simulink model "closed_loop_system_monitoring"  (R2025b)
settings: Solver=FixedStepAuto  StartTime=0.0  StopTime=2  RelTol=1e-3
values from neighbouring files (symbols this model uses):
  A = [Ac 0*Ac ... (first row only)    [closed_loop_system.m]
  B = [Bc ... (first row only)    [closed_loop_system.m]
  C = [0 0 Cp]    [closed_loop_system.m]
  Ts = 1/100    (= 0.01)    [closed_loop_system.m]
(part 2 of 2)

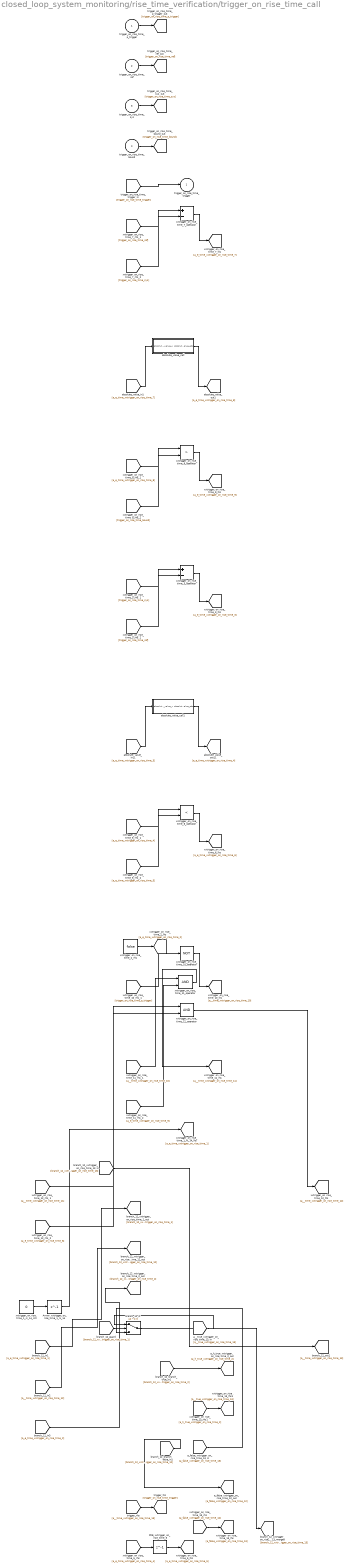
== system closed_loop_system_monitoring/rise_time_verification/trigger_on_rise_time_call ==
  trigger_on_rise_time_p_trigger : Inport  OutDataTypeStr=boolean
  trigger_on_rise_time_ref : Inport  Port=2  OutDataTypeStr=double
  trigger_on_rise_time_sys : Inport  Port=3  OutDataTypeStr=double
  trigger_on_rise_time_bound : Inport  Port=4  OutDataTypeStr=double
  Arrow_xxtrigger_on_rise_time_1_ni_14 : Delay  DelayLength=1  InitialCondition=1
  PRE_xxtrigger_on_rise_time_5 : Delay  DelayLength=1  InitialCondition=0
  absolute_value_call : Subsystem
  absolute_value_call1 : Subsystem
  branch_12_IF : Switch  Criteria=u2 ~= 0  SaturateOnIntegerOverflow=off  InputSameDT=off
  xxtrigger_on_rise_time_10_operator : Logic  Operator=NOT  AllPortsSameDT=off  OutDataTypeStr=boolean
  xxtrigger_on_rise_time_11_operator : Logic  AllPortsSameDT=off  OutDataTypeStr=boolean
  xxtrigger_on_rise_time_12_operator : Logic  AllPortsSameDT=off  OutDataTypeStr=boolean
  xxtrigger_on_rise_time_1_ni_14_init : Constant  Value=0  OutDataTypeStr=boolean
  xxtrigger_on_rise_time_2_rhs : Constant  Value=false  OutDataTypeStr=boolean
  xxtrigger_on_rise_time_3_operator : Sum  Inputs=+-  OutDataTypeStr=double
  xxtrigger_on_rise_time_6_operator : RelationalOperator  Operator=<  OutDataTypeStr=boolean  RndMeth=Simplest  InputSameDT=off
  xxtrigger_on_rise_time_7_operator : Sum  Inputs=+-  OutDataTypeStr=double
  xxtrigger_on_rise_time_9_operator : RelationalOperator  Operator=>  OutDataTypeStr=boolean  RndMeth=Simplest  InputSameDT=off
  trigger_on_rise_time_trigger : Outport
  wires:
  PRE_xxtrigger_on_rise_time_5/1 -> [a_e_time_xxtrigger_on_rise_time_5]
  [a_e_time_xxtrigger_on_rise_time_4] -> PRE_xxtrigger_on_rise_time_5/1
  [a__time_xxtrigger_on_rise_time_13] -> [trigger_on_rise_time_trigger]
  [branch_12_xxtrigger_on_rise_time_2] -> [a_h_true_xxtrigger_on_rise_time_2]
  [a_h_true_xxtrigger_on_rise_time_2] -> [a__true_xxtrigger_on_rise_time_13]
  [branch_12_xxtrigger_on_rise_time_12] -> [a_false_xxtrigger_on_rise_time_12]
  [a_false_xxtrigger_on_rise_time_12] -> [a_false_xxtrigger_on_rise_time_13]
  [a_e_time_xxtrigger_on_rise_time_1] -> [branch_12_xxtrigger_on_rise_time_1]
  [a__time_xxtrigger_on_rise_time_12] -> [branch_12_xxtrigger_on_rise_time_12]
  [a_e_time_xxtrigger_on_rise_time_2] -> [branch_12_xxtrigger_on_rise_time_2]
  [branch_12_xxtrigger_on_rise_time_1] -> branch_12_IF/2
  [a__true_xxtrigger_on_rise_time_13] -> branch_12_IF/1
  [a_false_xxtrigger_on_rise_time_13] -> branch_12_IF/3
  branch_12_IF/1 -> [branch_12_xxtrigger_on_rise_time_13]
  [branch_12_xxtrigger_on_rise_time_13] -> [a__time_xxtrigger_on_rise_time_13]
  Arrow_xxtrigger_on_rise_time_1_ni_14/1 -> [a_e_time_xxtrigger_on_rise_time_1]
  xxtrigger_on_rise_time_1_ni_14_init/1 -> Arrow_xxtrigger_on_rise_time_1_ni_14/1
  [a_e_time_xxtrigger_on_rise_time_6] -> xxtrigger_on_rise_time_12_operator/2
  [a__time_xxtrigger_on_rise_time_11] -> xxtrigger_on_rise_time_12_operator/1
  xxtrigger_on_rise_time_12_operator/1 -> [a__time_xxtrigger_on_rise_time_12]
  [a_e_time_xxtrigger_on_rise_time_9] -> xxtrigger_on_rise_time_11_operator/2
  [a__time_xxtrigger_on_rise_time_10] -> xxtrigger_on_rise_time_11_operator/1
  xxtrigger_on_rise_time_11_operator/1 -> [a__time_xxtrigger_on_rise_time_11]
  [trigger_on_rise_time_p_trigger] -> xxtrigger_on_rise_time_10_operator/1
  xxtrigger_on_rise_time_10_operator/1 -> [a__time_xxtrigger_on_rise_time_10]
  xxtrigger_on_rise_time_2_rhs/1 -> [a_e_time_xxtrigger_on_rise_time_2]
  [a_e_time_xxtrigger_on_rise_time_5] -> xxtrigger_on_rise_time_6_operator/2
  [a_e_time_xxtrigger_on_rise_time_4] -> xxtrigger_on_rise_time_6_operator/1
  xxtrigger_on_rise_time_6_operator/1 -> [a_e_time_xxtrigger_on_rise_time_6]
  [a_e_time_xxtrigger_on_rise_time_3] -> absolute_value_call1/1(absolute_value_x)
  absolute_value_call1/1(absolute_value_abs) -> [a_e_time_xxtrigger_on_rise_time_4]
  [trigger_on_rise_time_ref] -> xxtrigger_on_rise_time_3_operator/2
  [trigger_on_rise_time_sys] -> xxtrigger_on_rise_time_3_operator/1
  xxtrigger_on_rise_time_3_operator/1 -> [a_e_time_xxtrigger_on_rise_time_3]
  [trigger_on_rise_time_bound] -> xxtrigger_on_rise_time_9_operator/2
  [a_e_time_xxtrigger_on_rise_time_8] -> xxtrigger_on_rise_time_9_operator/1
  xxtrigger_on_rise_time_9_operator/1 -> [a_e_time_xxtrigger_on_rise_time_9]
  [a_e_time_xxtrigger_on_rise_time_7] -> absolute_value_call/1(absolute_value_x)
  absolute_value_call/1(absolute_value_abs) -> [a_e_time_xxtrigger_on_rise_time_8]
  [trigger_on_rise_time_sys] -> xxtrigger_on_rise_time_7_operator/2
  [trigger_on_rise_time_ref] -> xxtrigger_on_rise_time_7_operator/1
  xxtrigger_on_rise_time_7_operator/1 -> [a_e_time_xxtrigger_on_rise_time_7]
  [trigger_on_rise_time_trigger] -> trigger_on_rise_time_trigger/1
  trigger_on_rise_time_bound/1 -> [trigger_on_rise_time_bound]
  trigger_on_rise_time_sys/1 -> [trigger_on_rise_time_sys]
  trigger_on_rise_time_ref/1 -> [trigger_on_rise_time_ref]
  trigger_on_rise_time_p_trigger/1 -> [trigger_on_rise_time_p_trigger]

== system closed_loop_system_monitoring/rise_time_verification/eventually_false_var_call/forall_a_var_call ==
  forall_a_var_inside_time_interval : Inport  OutDataTypeStr=boolean
  forall_a_var_prop : Inport  Port=2  OutDataTypeStr=boolean
  exist_var_call : Subsystem
  output_operator : Logic  Operator=NOT  AllPortsSameDT=off  OutDataTypeStr=boolean
  xxforall_a_var_1_operator : Logic  Operator=NOT  AllPortsSameDT=off  OutDataTypeStr=boolean
  forall_a_var_output : Outport
  wires:
  forall_a_var_inside_time_interval/1 -> [forall_a_var_inside_time_interval]
  forall_a_var_prop/1 -> [forall_a_var_prop]
  [forall_a_var_output] -> forall_a_var_output/1
  xxforall_a_var_1_operator/1 -> [forall_a_var_xxforall_a_var_1]
  [forall_a_var_prop] -> xxforall_a_var_1_operator/1
  exist_var_call/1(exist_var_output) -> [forall_a_var_xxforall_a_var_2]
  [forall_a_var_inside_time_interval] -> exist_var_call/1(exist_var_inside_time_interval)
  [forall_a_var_xxforall_a_var_1] -> exist_var_call/2(exist_var_prop)
  output_operator/1 -> [forall_a_var_output]
  [forall_a_var_xxforall_a_var_2] -> output_operator/1

== system closed_loop_system_monitoring/rise_time_verification/eventually_false_var_call/min_call ==
  min_a : Inport
  min_b : Inport  Port=2
  branch_1_IF : Switch  Criteria=u2 ~= 0  SaturateOnIntegerOverflow=off  InputSameDT=off
  xxmin_1_operator : RelationalOperator  Operator=<=  OutDataTypeStr=boolean  RndMeth=Simplest  InputSameDT=off
  min_valeur_min : Outport
  wires:
  min_a/1 -> [min_a]
  min_b/1 -> [min_b]
  [min_valeur_min] -> min_valeur_min/1
  xxmin_1_operator/1 -> [min_xxmin_1]
  [min_a] -> xxmin_1_operator/1
  [min_b] -> xxmin_1_operator/2
  [branch_1_valeur_min] -> [min_valeur_min]
  branch_1_IF/1 -> [branch_1_valeur_min]
  [branch_1_branch_false_valeur_min] -> branch_1_IF/3
  [branch_1_branch_true_valeur_min] -> branch_1_IF/1
  [branch_1_xxmin_1] -> branch_1_IF/2
  [min_b] -> [branch_1_b]
  [min_a] -> [branch_1_a]
  [min_xxmin_1] -> [branch_1_xxmin_1]
  [branch_1_branch_false_b] -> [branch_1_branch_false_valeur_min]
  [branch_1_b] -> [branch_1_branch_false_b]
  [branch_1_branch_true_a] -> [branch_1_branch_true_valeur_min]
  [branch_1_a] -> [branch_1_branch_true_a]

== system closed_loop_system_monitoring/rise_time_verification/eventually_false_var_call/timeab_var_call ==
  timeab_var_a : Inport
  timeab_var_b : Inport  Port=2
  timeab_tmp_var_call : Subsystem
  timeab_var_inside_time_interval : Outport
  wires:
  timeab_var_a/1 -> [timeab_var_a]
  timeab_var_b/1 -> [timeab_var_b]
  [timeab_var_inside_time_interval] -> timeab_var_inside_time_interval/1
  timeab_tmp_var_call/1(timeab_tmp_var_internal_clk) -> [timeab_var_iclk]
  timeab_tmp_var_call/2(timeab_tmp_var_inside_time_interval) -> [timeab_var_inside_time_interval]
  [timeab_var_a] -> timeab_tmp_var_call/1(timeab_tmp_var_a)
  [timeab_var_b] -> timeab_tmp_var_call/2(timeab_tmp_var_b)

== system closed_loop_system_monitoring/rise_time_verification/eventually_true_var_call/exist_var_call ==
  exist_var_inside_time_interval : Inport  OutDataTypeStr=boolean
  exist_var_prop : Inport  Port=2  OutDataTypeStr=boolean
  output_operator : Logic  AllPortsSameDT=off  OutDataTypeStr=boolean
  exist_var_output : Outport
  wires:
  exist_var_inside_time_interval/1 -> [exist_var_inside_time_interval]
  exist_var_prop/1 -> [exist_var_prop]
  [exist_var_output] -> exist_var_output/1
  output_operator/1 -> [exist_var_output]
  [exist_var_inside_time_interval] -> output_operator/1
  [exist_var_prop] -> output_operator/2

== system closed_loop_system_monitoring/rise_time_verification/eventually_true_var_call/timeab_var_call ==
  timeab_var_a : Inport
  timeab_var_b : Inport  Port=2
  Scope : Scope  NumInputPorts=4
      settings: ActiveDisplayYMinimum=-0.12499999999999997  ActiveDisplayYMaximum=1.125  DataLoggingVariableName=ScopeData12
  timeab_tmp_var_call : Subsystem
  timeab_var_inside_time_interval : Outport
  wires:
  timeab_var_a/1 -> [timeab_var_a]
  timeab_var_b/1 -> [timeab_var_b]
  [timeab_var_inside_time_interval] -> timeab_var_inside_time_interval/1
  timeab_tmp_var_call/1(timeab_tmp_var_internal_clk) -> Scope/2, [timeab_var_iclk]
  timeab_tmp_var_call/2(timeab_tmp_var_inside_time_interval) -> Scope/1, [timeab_var_inside_time_interval]
  [timeab_var_a] -> Scope/3, timeab_tmp_var_call/1(timeab_tmp_var_a)
  [timeab_var_b] -> timeab_tmp_var_call/2(timeab_tmp_var_b), Scope/4

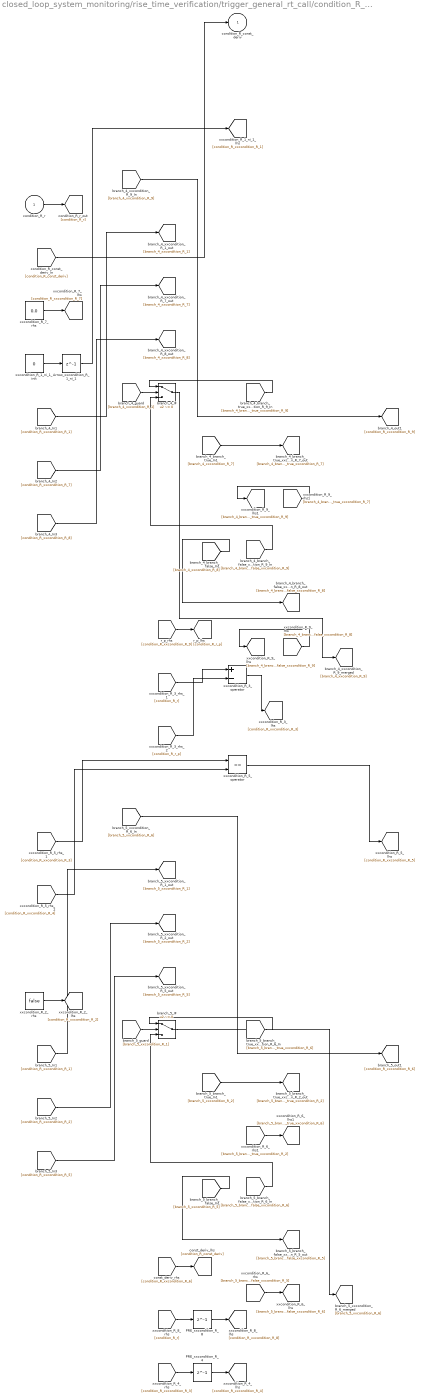
== system closed_loop_system_monitoring/rise_time_verification/trigger_general_rt_call/condition_R_call ==
  condition_R_r : Inport  OutDataTypeStr=double
  Arrow_xxcondition_R_1_ni_1 : Delay  DelayLength=1  InitialCondition=1
  PRE_xxcondition_R_4 : Delay  DelayLength=1  InitialCondition=0
  PRE_xxcondition_R_8 : Delay  DelayLength=1  InitialCondition=0
  branch_4_IF : Switch  Criteria=u2 ~= 0  SaturateOnIntegerOverflow=off  InputSameDT=off
  branch_5_IF : Switch  Criteria=u2 ~= 0  SaturateOnIntegerOverflow=off  InputSameDT=off
  xxcondition_R_1_ni_1_init : Constant  Value=0  OutDataTypeStr=boolean
  xxcondition_R_2_rhs : Constant  Value=false  OutDataTypeStr=boolean
  xxcondition_R_3_operator : Sum  Inputs=+-  OutDataTypeStr=double
  xxcondition_R_5_operator : RelationalOperator  Operator===  OutDataTypeStr=boolean  RndMeth=Simplest  InputSameDT=off
  xxcondition_R_7_rhs : Constant  Value=0.0  OutDataTypeStr=double
  condition_R_const_deriv : Outport
  wires:
  condition_R_r/1 -> [condition_R_r]
  [condition_R_const_deriv] -> condition_R_const_deriv/1
  xxcondition_R_7_rhs/1 -> [condition_R_xxcondition_R_7]
  xxcondition_R_1_ni_1_init/1 -> Arrow_xxcondition_R_1_ni_1/1
  Arrow_xxcondition_R_1_ni_1/1 -> [condition_R_xxcondition_R_1]
  [branch_4_xxcondition_R_9] -> [condition_R_xxcondition_R_9]
  branch_4_IF/1 -> [branch_4_xxcondition_R_9]
  [branch_4_branch_false_xxcondition_R_9] -> branch_4_IF/3
  [branch_4_branch_true_xxcondition_R_9] -> branch_4_IF/1
  [branch_4_xxcondition_R_1] -> branch_4_IF/2
  [condition_R_xxcondition_R_8] -> [branch_4_xxcondition_R_8]
  [condition_R_xxcondition_R_7] -> [branch_4_xxcondition_R_7]
  [condition_R_xxcondition_R_1] -> [branch_4_xxcondition_R_1]
  [branch_4_branch_false_xxcondition_R_8] -> [branch_4_branch_false_xxcondition_R_9]
  [branch_4_xxcondition_R_8] -> [branch_4_branch_false_xxcondition_R_8]
  [branch_4_branch_true_xxcondition_R_7] -> [branch_4_branch_true_xxcondition_R_9]
  [branch_4_xxcondition_R_7] -> [branch_4_branch_true_xxcondition_R_7]
  [condition_R_xxcondition_R_9] -> [condition_R_r_p]
  xxcondition_R_3_operator/1 -> [condition_R_xxcondition_R_3]
  [condition_R_r] -> xxcondition_R_3_operator/1
  [condition_R_r_p] -> xxcondition_R_3_operator/2
  xxcondition_R_5_operator/1 -> [condition_R_xxcondition_R_5]
  [condition_R_xxcondition_R_3] -> xxcondition_R_5_operator/1
  [condition_R_xxcondition_R_4] -> xxcondition_R_5_operator/2
  xxcondition_R_2_rhs/1 -> [condition_R_xxcondition_R_2]
  [branch_5_xxcondition_R_6] -> [condition_R_xxcondition_R_6]
  branch_5_IF/1 -> [branch_5_xxcondition_R_6]
  [branch_5_branch_false_xxcondition_R_6] -> branch_5_IF/3
  [branch_5_branch_true_xxcondition_R_6] -> branch_5_IF/1
  [branch_5_xxcondition_R_1] -> branch_5_IF/2
  [condition_R_xxcondition_R_5] -> [branch_5_xxcondition_R_5]
  [condition_R_xxcondition_R_2] -> [branch_5_xxcondition_R_2]
  [condition_R_xxcondition_R_1] -> [branch_5_xxcondition_R_1]
  [branch_5_branch_false_xxcondition_R_5] -> [branch_5_branch_false_xxcondition_R_6]
  [branch_5_xxcondition_R_5] -> [branch_5_branch_false_xxcondition_R_5]
  [branch_5_branch_true_xxcondition_R_2] -> [branch_5_branch_true_xxcondition_R_6]
  [branch_5_xxcondition_R_2] -> [branch_5_branch_true_xxcondition_R_2]
  [condition_R_xxcondition_R_6] -> [condition_R_const_deriv]
  [condition_R_r] -> PRE_xxcondition_R_8/1
  PRE_xxcondition_R_8/1 -> [condition_R_xxcondition_R_8]
  [condition_R_xxcondition_R_3] -> PRE_xxcondition_R_4/1
  PRE_xxcondition_R_4/1 -> [condition_R_xxcondition_R_4]

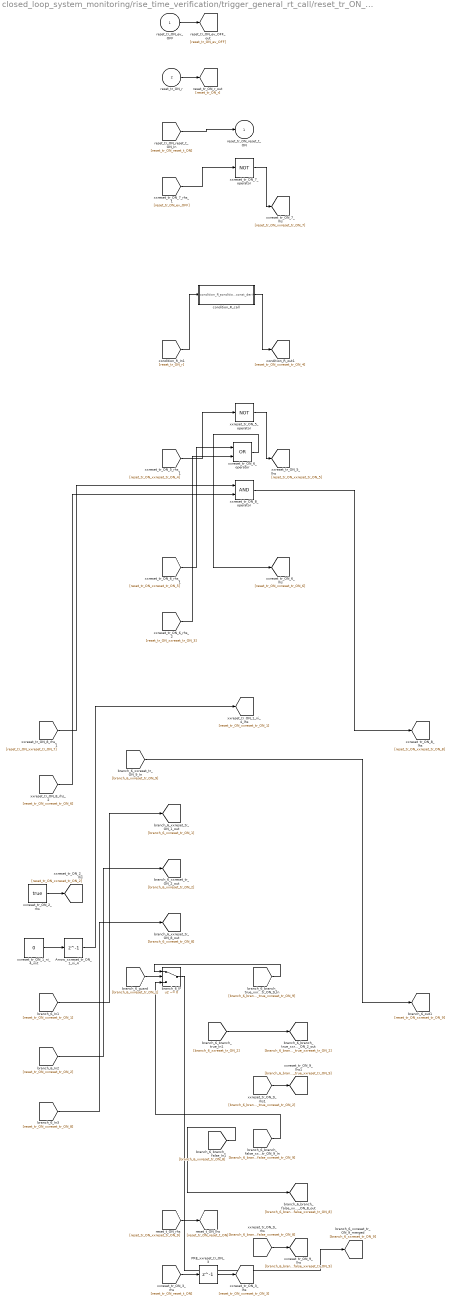
== system closed_loop_system_monitoring/rise_time_verification/trigger_general_rt_call/reset_tr_ON_call ==
  reset_tr_ON_ev_OFF : Inport  OutDataTypeStr=boolean
  reset_tr_ON_r : Inport  Port=2  OutDataTypeStr=double
  Arrow_xxreset_tr_ON_1_ni_4 : Delay  DelayLength=1  InitialCondition=1
  PRE_xxreset_tr_ON_3 : Delay  DelayLength=1  InitialCondition=0
  branch_6_IF : Switch  Criteria=u2 ~= 0  SaturateOnIntegerOverflow=off  InputSameDT=off
  condition_R_call : Subsystem
  xxreset_tr_ON_1_ni_4_init : Constant  Value=0  OutDataTypeStr=boolean
  xxreset_tr_ON_2_rhs : Constant  Value=true  OutDataTypeStr=boolean
  xxreset_tr_ON_5_operator : Logic  Operator=NOT  AllPortsSameDT=off  OutDataTypeStr=boolean
  xxreset_tr_ON_6_operator : Logic  Operator=OR  AllPortsSameDT=off  OutDataTypeStr=boolean
  xxreset_tr_ON_7_operator : Logic  Operator=NOT  AllPortsSameDT=off  OutDataTypeStr=boolean
  xxreset_tr_ON_8_operator : Logic  AllPortsSameDT=off  OutDataTypeStr=boolean
  reset_tr_ON_reset_t_ON : Outport
  wires:
  reset_tr_ON_ev_OFF/1 -> [reset_tr_ON_ev_OFF]
  reset_tr_ON_r/1 -> [reset_tr_ON_r]
  [reset_tr_ON_reset_t_ON] -> reset_tr_ON_reset_t_ON/1
  xxreset_tr_ON_7_operator/1 -> [reset_tr_ON_xxreset_tr_ON_7]
  [reset_tr_ON_ev_OFF] -> xxreset_tr_ON_7_operator/1
  condition_R_call/1(condition_R_const_deriv) -> [reset_tr_ON_xxreset_tr_ON_4]
  [reset_tr_ON_r] -> condition_R_call/1(condition_R_r)
  xxreset_tr_ON_5_operator/1 -> [reset_tr_ON_xxreset_tr_ON_5]
  [reset_tr_ON_xxreset_tr_ON_4] -> xxreset_tr_ON_5_operator/1
  xxreset_tr_ON_6_operator/1 -> [reset_tr_ON_xxreset_tr_ON_6]
  [reset_tr_ON_xxreset_tr_ON_5] -> xxreset_tr_ON_6_operator/1
  [reset_tr_ON_xxreset_tr_ON_3] -> xxreset_tr_ON_6_operator/2
  xxreset_tr_ON_8_operator/1 -> [reset_tr_ON_xxreset_tr_ON_8]
  [reset_tr_ON_xxreset_tr_ON_7] -> xxreset_tr_ON_8_operator/1
  [reset_tr_ON_xxreset_tr_ON_6] -> xxreset_tr_ON_8_operator/2
  xxreset_tr_ON_2_rhs/1 -> [reset_tr_ON_xxreset_tr_ON_2]
  xxreset_tr_ON_1_ni_4_init/1 -> Arrow_xxreset_tr_ON_1_ni_4/1
  Arrow_xxreset_tr_ON_1_ni_4/1 -> [reset_tr_ON_xxreset_tr_ON_1]
  [branch_6_xxreset_tr_ON_9] -> [reset_tr_ON_xxreset_tr_ON_9]
  branch_6_IF/1 -> [branch_6_xxreset_tr_ON_9]
  [branch_6_branch_false_xxreset_tr_ON_9] -> branch_6_IF/3
  [branch_6_branch_true_xxreset_tr_ON_9] -> branch_6_IF/1
  [branch_6_xxreset_tr_ON_1] -> branch_6_IF/2
  [reset_tr_ON_xxreset_tr_ON_8] -> [branch_6_xxreset_tr_ON_8]
  [reset_tr_ON_xxreset_tr_ON_2] -> [branch_6_xxreset_tr_ON_2]
  [reset_tr_ON_xxreset_tr_ON_1] -> [branch_6_xxreset_tr_ON_1]
  [branch_6_branch_false_xxreset_tr_ON_8] -> [branch_6_branch_false_xxreset_tr_ON_9]
  [branch_6_xxreset_tr_ON_8] -> [branch_6_branch_false_xxreset_tr_ON_8]
  [branch_6_branch_true_xxreset_tr_ON_2] -> [branch_6_branch_true_xxreset_tr_ON_9]
  [branch_6_xxreset_tr_ON_2] -> [branch_6_branch_true_xxreset_tr_ON_2]
  [reset_tr_ON_xxreset_tr_ON_9] -> [reset_tr_ON_reset_t_ON]
  [reset_tr_ON_reset_t_ON] -> PRE_xxreset_tr_ON_3/1
  PRE_xxreset_tr_ON_3/1 -> [reset_tr_ON_xxreset_tr_ON_3]

== system closed_loop_system_monitoring/rise_time_verification/trigger_general_rt_call/since_call ==
  since_ev_ON : Inport  OutDataTypeStr=boolean
  since_ev_OFF : Inport  Port=2  OutDataTypeStr=boolean
  Arrow_xxsince_1_ni_5 : Delay  DelayLength=1  InitialCondition=1
  branch_7_IF : Switch  Criteria=u2 ~= 0  SaturateOnIntegerOverflow=off  InputSameDT=off
  xxsince_1_ni_5_init : Constant  Value=0  OutDataTypeStr=boolean
  xxsince_2_operator : Logic  Operator=NOT  AllPortsSameDT=off  OutDataTypeStr=boolean
  xxsince_3_operator : Logic  AllPortsSameDT=off  OutDataTypeStr=boolean
  since_out : Outport
  wires:
  since_ev_ON/1 -> [since_ev_ON]
  since_ev_OFF/1 -> [since_ev_OFF]
  [since_out] -> since_out/1
  xxsince_2_operator/1 -> [since_xxsince_2]
  [since_ev_OFF] -> xxsince_2_operator/1
  xxsince_3_operator/1 -> [since_xxsince_3]
  [since_ev_ON] -> xxsince_3_operator/1
  [since_xxsince_2] -> xxsince_3_operator/2
  xxsince_1_ni_5_init/1 -> Arrow_xxsince_1_ni_5/1
  Arrow_xxsince_1_ni_5/1 -> [since_xxsince_1]
  [branch_7_xxsince_4] -> [since_xxsince_4]
  branch_7_IF/1 -> [branch_7_xxsince_4]
  [branch_7_branch_false_xxsince_4] -> branch_7_IF/3
  [branch_7_branch_true_xxsince_4] -> branch_7_IF/1
  [branch_7_xxsince_1] -> branch_7_IF/2
  [since_ev_ON] -> [branch_7_ev_ON]
  [since_xxsince_3] -> [branch_7_xxsince_3]
  [since_xxsince_1] -> [branch_7_xxsince_1]
  [branch_7_branch_false_xxsince_3] -> [branch_7_branch_false_xxsince_4]
  [branch_7_xxsince_3] -> [branch_7_branch_false_xxsince_3]
  [branch_7_branch_true_ev_ON] -> [branch_7_branch_true_xxsince_4]
  [branch_7_ev_ON] -> [branch_7_branch_true_ev_ON]
  [since_xxsince_4] -> [since_out]

== system closed_loop_system_monitoring/rise_time_verification/trigger_off_rise_time_call/absolute_value_call ==
  absolute_value_x : Inport  OutDataTypeStr=double
  branch_8_IF : Switch  Criteria=u2 ~= 0  SaturateOnIntegerOverflow=off  InputSameDT=off
  xxabsolute_value_1_operator : RelationalOperator  OutDataTypeStr=boolean  RndMeth=Simplest  InputSameDT=off
  xxabsolute_value_1_rhs_2 : Constant  Value=0.0  OutDataTypeStr=double
  xxabsolute_value_2_operator : Gain  Gain=-1  OutDataTypeStr=double
  absolute_value_abs : Outport
  wires:
  absolute_value_x/1 -> [absolute_value_x]
  [absolute_value_abs] -> absolute_value_abs/1
  xxabsolute_value_2_operator/1 -> [absolute_value_xxabsolute_value_2]
  [absolute_value_x] -> xxabsolute_value_2_operator/1
  xxabsolute_value_1_operator/1 -> [absolute_value_xxabsolute_value_1]
  [absolute_value_x] -> xxabsolute_value_1_operator/1
  xxabsolute_value_1_rhs_2/1 -> xxabsolute_value_1_operator/2
  [branch_8_abs] -> [absolute_value_abs]
  branch_8_IF/1 -> [branch_8_abs]
  [branch_8_branch_false_abs] -> branch_8_IF/3
  [branch_8_branch_true_abs] -> branch_8_IF/1
  [branch_8_xxabsolute_value_1] -> branch_8_IF/2
  [absolute_value_x] -> [branch_8_x]
  [absolute_value_xxabsolute_value_2] -> [branch_8_xxabsolute_value_2]
  [absolute_value_xxabsolute_value_1] -> [branch_8_xxabsolute_value_1]
  [branch_8_branch_false_xxabsolute_value_2] -> [branch_8_branch_false_abs]
  [branch_8_xxabsolute_value_2] -> [branch_8_branch_false_xxabsolute_value_2]
  [branch_8_branch_true_x] -> [branch_8_branch_true_abs]
  [branch_8_x] -> [branch_8_branch_true_x]

== system closed_loop_system_monitoring/rise_time_verification/trigger_on_rise_time_call/absolute_value_call ==
  absolute_value_x : Inport  OutDataTypeStr=double
  branch_8_IF : Switch  Criteria=u2 ~= 0  SaturateOnIntegerOverflow=off  InputSameDT=off
  xxabsolute_value_1_operator : RelationalOperator  OutDataTypeStr=boolean  RndMeth=Simplest  InputSameDT=off
  xxabsolute_value_1_rhs_2 : Constant  Value=0.0  OutDataTypeStr=double
  xxabsolute_value_2_operator : Gain  Gain=-1  OutDataTypeStr=double
  absolute_value_abs : Outport
  wires:
  absolute_value_x/1 -> [absolute_value_x]
  [absolute_value_abs] -> absolute_value_abs/1
  xxabsolute_value_2_operator/1 -> [absolute_value_xxabsolute_value_2]
  [absolute_value_x] -> xxabsolute_value_2_operator/1
  xxabsolute_value_1_operator/1 -> [absolute_value_xxabsolute_value_1]
  [absolute_value_x] -> xxabsolute_value_1_operator/1
  xxabsolute_value_1_rhs_2/1 -> xxabsolute_value_1_operator/2
  [branch_8_abs] -> [absolute_value_abs]
  branch_8_IF/1 -> [branch_8_abs]
  [branch_8_branch_false_abs] -> branch_8_IF/3
  [branch_8_branch_true_abs] -> branch_8_IF/1
  [branch_8_xxabsolute_value_1] -> branch_8_IF/2
  [absolute_value_x] -> [branch_8_x]
  [absolute_value_xxabsolute_value_2] -> [branch_8_xxabsolute_value_2]
  [absolute_value_xxabsolute_value_1] -> [branch_8_xxabsolute_value_1]
  [branch_8_branch_false_xxabsolute_value_2] -> [branch_8_branch_false_abs]
  [branch_8_xxabsolute_value_2] -> [branch_8_branch_false_xxabsolute_value_2]
  [branch_8_branch_true_x] -> [branch_8_branch_true_abs]
  [branch_8_x] -> [branch_8_branch_true_x]

== system closed_loop_system_monitoring/rise_time_verification/trigger_on_rise_time_call/absolute_value_call1 ==
  absolute_value_x : Inport  OutDataTypeStr=double
  branch_8_IF : Switch  Criteria=u2 ~= 0  SaturateOnIntegerOverflow=off  InputSameDT=off
  xxabsolute_value_1_operator : RelationalOperator  OutDataTypeStr=boolean  RndMeth=Simplest  InputSameDT=off
  xxabsolute_value_1_rhs_2 : Constant  Value=0.0  OutDataTypeStr=double
  xxabsolute_value_2_operator : Gain  Gain=-1  OutDataTypeStr=double
  absolute_value_abs : Outport
  wires:
  absolute_value_x/1 -> [absolute_value_x]
  [absolute_value_abs] -> absolute_value_abs/1
  xxabsolute_value_2_operator/1 -> [absolute_value_xxabsolute_value_2]
  [absolute_value_x] -> xxabsolute_value_2_operator/1
  xxabsolute_value_1_operator/1 -> [absolute_value_xxabsolute_value_1]
  [absolute_value_x] -> xxabsolute_value_1_operator/1
  xxabsolute_value_1_rhs_2/1 -> xxabsolute_value_1_operator/2
  [branch_8_abs] -> [absolute_value_abs]
  branch_8_IF/1 -> [branch_8_abs]
  [branch_8_branch_false_abs] -> branch_8_IF/3
  [branch_8_branch_true_abs] -> branch_8_IF/1
  [branch_8_xxabsolute_value_1] -> branch_8_IF/2
  [absolute_value_x] -> [branch_8_x]
  [absolute_value_xxabsolute_value_2] -> [branch_8_xxabsolute_value_2]
  [absolute_value_xxabsolute_value_1] -> [branch_8_xxabsolute_value_1]
  [branch_8_branch_false_xxabsolute_value_2] -> [branch_8_branch_false_abs]
  [branch_8_xxabsolute_value_2] -> [branch_8_branch_false_xxabsolute_value_2]
  [branch_8_branch_true_x] -> [branch_8_branch_true_abs]
  [branch_8_x] -> [branch_8_branch_true_x]

== system closed_loop_system_monitoring/rise_time_verification/eventually_false_var_call/forall_a_var_call/exist_var_call ==
  exist_var_inside_time_interval : Inport  OutDataTypeStr=boolean
  exist_var_prop : Inport  Port=2  OutDataTypeStr=boolean
  output_operator : Logic  AllPortsSameDT=off  OutDataTypeStr=boolean
  exist_var_output : Outport
  wires:
  [exist_var_prop] -> output_operator/2
  [exist_var_inside_time_interval] -> output_operator/1
  output_operator/1 -> [exist_var_output]
  [exist_var_output] -> exist_var_output/1
  exist_var_prop/1 -> [exist_var_prop]
  exist_var_inside_time_interval/1 -> [exist_var_inside_time_interval]

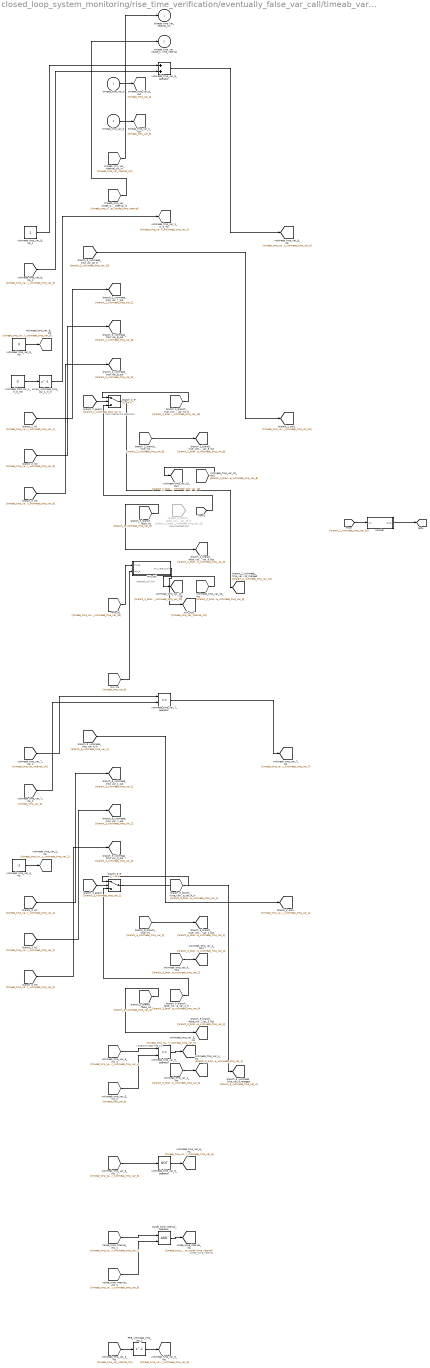
== system closed_loop_system_monitoring/rise_time_verification/eventually_false_var_call/timeab_var_call/timeab_tmp_var_call ==
  note: I SUBSTITUTED THE ==
  note: Internal_clk min
  note: INIT internal clk
      | Guard OK
  note: Inside_time_interval
  timeab_tmp_var_a : Inport
  timeab_tmp_var_b : Inport  Port=2
  Arrow_xxtimeab_tmp_var_1_ni_0 : Delay  DelayLength=1  InitialCondition=1
  PRE_xxtimeab_tmp_var_3 : Delay  DelayLength=1  InitialCondition=0
  branch_2_IF : Switch  Criteria=u2 ~= 0  SaturateOnIntegerOverflow=off  InputSameDT=off
  branch_2_branch_false_xxtimeab_tmp_var_10_In : From  Commented=on  GotoTag=branch_2_branch_false_xxtimeab_tmp_var_10
  branch_3_IF : Switch  Criteria=u2 ~= 0  SaturateOnIntegerOverflow=off  InputSameDT=off
  counter : Subsystem
  inside_time_interval_operator : Logic  AllPortsSameDT=off  OutDataTypeStr=boolean
  min_call : Subsystem
  xxtimeab_tmp_var_1_ni_0_init : Constant  Value=0  OutDataTypeStr=boolean
  xxtimeab_tmp_var_2_rhs : Constant  Value=-1  OutDataTypeStr=Inherit: Inherit via back propagation
  xxtimeab_tmp_var_5_operator : RelationalOperator  OutDataTypeStr=boolean  RndMeth=Simplest  InputSameDT=off
  xxtimeab_tmp_var_6_operator : Logic  Operator=NOT  AllPortsSameDT=off  OutDataTypeStr=boolean
  xxtimeab_tmp_var_7_operator : RelationalOperator  OutDataTypeStr=boolean  RndMeth=Simplest  InputSameDT=off
  xxtimeab_tmp_var_8_rhs : Constant  Value=0  OutDataTypeStr=Inherit: Inherit via back propagation
  xxtimeab_tmp_var_9_operator : Sum  OutDataTypeStr=int32
  xxtimeab_tmp_var_9_rhs_1 : Constant  OutDataTypeStr=int32
  timeab_tmp_var_internal_clk : Outport
  timeab_tmp_var_inside_time_interval : Outport  Port=2
  wires:
  PRE_xxtimeab_tmp_var_3/1 -> [timeab_tmp_var_xxtimeab_tmp_var_3]
  [timeab_tmp_var_internal_clk] -> PRE_xxtimeab_tmp_var_3/1
  [timeab_tmp_var_xxtimeab_tmp_var_6] -> inside_time_interval_operator/2
  [timeab_tmp_var_xxtimeab_tmp_var_7] -> inside_time_interval_operator/1
  inside_time_interval_operator/1 -> [timeab_tmp_var_inside_time_interval]
  [timeab_tmp_var_xxtimeab_tmp_var_5] -> xxtimeab_tmp_var_6_operator/1
  xxtimeab_tmp_var_6_operator/1 -> [timeab_tmp_var_xxtimeab_tmp_var_6]
  [timeab_tmp_var_b] -> xxtimeab_tmp_var_5_operator/2
  [timeab_tmp_var_xxtimeab_tmp_var_4] -> xxtimeab_tmp_var_5_operator/1
  xxtimeab_tmp_var_5_operator/1 -> [timeab_tmp_var_xxtimeab_tmp_var_5]
  [branch_3_xxtimeab_tmp_var_2] -> [branch_3_branch_true_xxtimeab_tmp_var_2]
  [branch_3_branch_true_xxtimeab_tmp_var_2] -> [branch_3_branch_true_xxtimeab_tmp_var_4]
  [branch_3_xxtimeab_tmp_var_3] -> [branch_3_branch_false_xxtimeab_tmp_var_3]
  [branch_3_branch_false_xxtimeab_tmp_var_3] -> [branch_3_branch_false_xxtimeab_tmp_var_4]
  [timeab_tmp_var_xxtimeab_tmp_var_1] -> [branch_3_xxtimeab_tmp_var_1]
  [timeab_tmp_var_xxtimeab_tmp_var_2] -> [branch_3_xxtimeab_tmp_var_2]
  [timeab_tmp_var_xxtimeab_tmp_var_3] -> [branch_3_xxtimeab_tmp_var_3]
  [branch_3_xxtimeab_tmp_var_1] -> branch_3_IF/2
  [branch_3_branch_true_xxtimeab_tmp_var_4] -> branch_3_IF/1
  [branch_3_branch_false_xxtimeab_tmp_var_4] -> branch_3_IF/3
  branch_3_IF/1 -> [branch_3_xxtimeab_tmp_var_4]
  [branch_3_xxtimeab_tmp_var_4] -> [timeab_tmp_var_xxtimeab_tmp_var_4]
  xxtimeab_tmp_var_2_rhs/1 -> [timeab_tmp_var_xxtimeab_tmp_var_2]
  [timeab_tmp_var_a] -> xxtimeab_tmp_var_7_operator/2
  [timeab_tmp_var_internal_clk] -> xxtimeab_tmp_var_7_operator/1
  xxtimeab_tmp_var_7_operator/1 -> [timeab_tmp_var_xxtimeab_tmp_var_7]
  [timeab_tmp_var_b] -> min_call/2(min_b)
  [timeab_tmp_var_xxtimeab_tmp_var_10] -> min_call/1(min_a)
  min_call/1(min_valeur_min) -> [timeab_tmp_var_internal_clk]
  [branch_2_xxtimeab_tmp_var_8] -> [branch_2_branch_true_xxtimeab_tmp_var_8]
  [branch_2_branch_true_xxtimeab_tmp_var_8] -> [branch_2_branch_true_xxtimeab_tmp_var_10]
  [branch_2_xxtimeab_tmp_var_9] -> [branch_2_branch_false_xxtimeab_tmp_var_9]
  [branch_2_branch_false_xxtimeab_tmp_var_9] -> [branch_2_branch_false_xxtimeab_tmp_var_10]
  [timeab_tmp_var_xxtimeab_tmp_var_1] -> [branch_2_xxtimeab_tmp_var_1]
  [timeab_tmp_var_xxtimeab_tmp_var_8] -> [branch_2_xxtimeab_tmp_var_8]
  [timeab_tmp_var_xxtimeab_tmp_var_9] -> [branch_2_xxtimeab_tmp_var_9]
  [branch_2_xxtimeab_tmp_var_1] -> branch_2_IF/2
  [branch_2_branch_true_xxtimeab_tmp_var_10] -> branch_2_IF/1
  [Counter] -> branch_2_IF/3
  branch_2_IF/1 -> [branch_2_xxtimeab_tmp_var_10]
  [branch_2_xxtimeab_tmp_var_10] -> [timeab_tmp_var_xxtimeab_tmp_var_10]
  Arrow_xxtimeab_tmp_var_1_ni_0/1 -> [timeab_tmp_var_xxtimeab_tmp_var_1]
  xxtimeab_tmp_var_1_ni_0_init/1 -> Arrow_xxtimeab_tmp_var_1_ni_0/1
  xxtimeab_tmp_var_8_rhs/1 -> [timeab_tmp_var_xxtimeab_tmp_var_8]
  [timeab_tmp_var_xxtimeab_tmp_var_3] -> xxtimeab_tmp_var_9_operator/2
  xxtimeab_tmp_var_9_rhs_1/1 -> xxtimeab_tmp_var_9_operator/1
  xxtimeab_tmp_var_9_operator/1 -> [timeab_tmp_var_xxtimeab_tmp_var_9]
  [timeab_tmp_var_inside_time_interval] -> timeab_tmp_var_inside_time_interval/1
  [timeab_tmp_var_internal_clk] -> timeab_tmp_var_internal_clk/1
  timeab_tmp_var_b/1 -> [timeab_tmp_var_b]
  timeab_tmp_var_a/1 -> [timeab_tmp_var_a]
  [branch_2_xxtimeab_tmp_var_10] -> counter/1(In1)
  counter/1(Out1) -> [Counter]

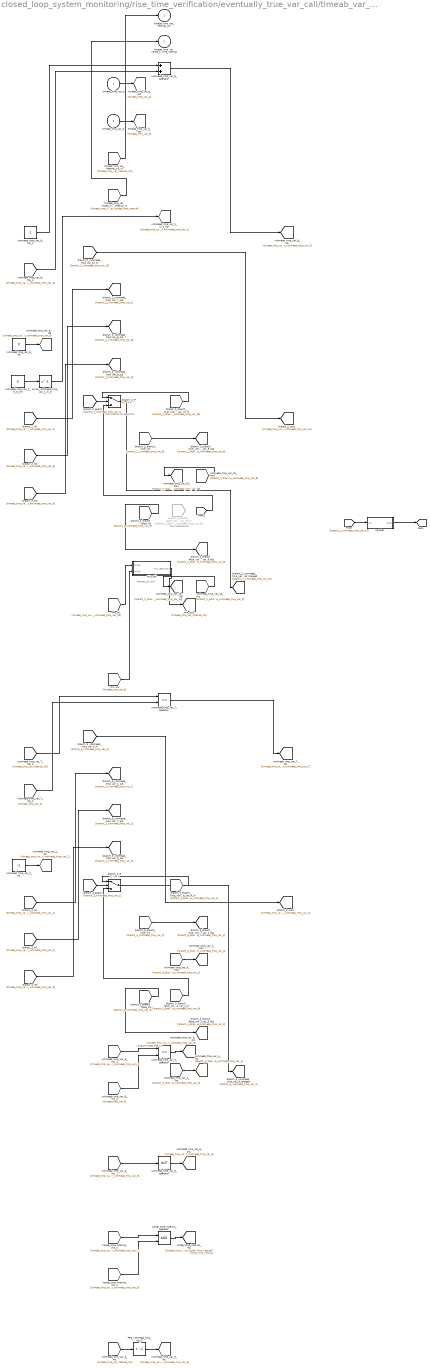
== system closed_loop_system_monitoring/rise_time_verification/eventually_true_var_call/timeab_var_call/timeab_tmp_var_call ==
  note: I SUBSTITUTED THE ==
  note: Internal_clk min
  note: INIT internal clk
      | Guard OK
  note: Inside_time_interval
  timeab_tmp_var_a : Inport
  timeab_tmp_var_b : Inport  Port=2
  Arrow_xxtimeab_tmp_var_1_ni_0 : Delay  DelayLength=1  InitialCondition=1
  PRE_xxtimeab_tmp_var_3 : Delay  DelayLength=1  InitialCondition=0
  branch_2_IF : Switch  Criteria=u2 ~= 0  SaturateOnIntegerOverflow=off  InputSameDT=off
  branch_2_branch_false_xxtimeab_tmp_var_10_In : From  Commented=on  GotoTag=branch_2_branch_false_xxtimeab_tmp_var_10
  branch_3_IF : Switch  Criteria=u2 ~= 0  SaturateOnIntegerOverflow=off  InputSameDT=off
  counter : Subsystem
  inside_time_interval_operator : Logic  AllPortsSameDT=off  OutDataTypeStr=boolean
  min_call : Subsystem
  xxtimeab_tmp_var_1_ni_0_init : Constant  Value=0  OutDataTypeStr=boolean
  xxtimeab_tmp_var_2_rhs : Constant  Value=-1  OutDataTypeStr=Inherit: Inherit via back propagation
  xxtimeab_tmp_var_5_operator : RelationalOperator  OutDataTypeStr=boolean  RndMeth=Simplest  InputSameDT=off
  xxtimeab_tmp_var_6_operator : Logic  Operator=NOT  AllPortsSameDT=off  OutDataTypeStr=boolean
  xxtimeab_tmp_var_7_operator : RelationalOperator  OutDataTypeStr=boolean  RndMeth=Simplest  InputSameDT=off
  xxtimeab_tmp_var_8_rhs : Constant  Value=0  OutDataTypeStr=Inherit: Inherit via back propagation
  xxtimeab_tmp_var_9_operator : Sum  OutDataTypeStr=int32
  xxtimeab_tmp_var_9_rhs_1 : Constant  OutDataTypeStr=int32
  timeab_tmp_var_internal_clk : Outport
  timeab_tmp_var_inside_time_interval : Outport  Port=2
  wires:
  PRE_xxtimeab_tmp_var_3/1 -> [timeab_tmp_var_xxtimeab_tmp_var_3]
  [timeab_tmp_var_internal_clk] -> PRE_xxtimeab_tmp_var_3/1
  [timeab_tmp_var_xxtimeab_tmp_var_6] -> inside_time_interval_operator/2
  [timeab_tmp_var_xxtimeab_tmp_var_7] -> inside_time_interval_operator/1
  inside_time_interval_operator/1 -> [timeab_tmp_var_inside_time_interval]
  [timeab_tmp_var_xxtimeab_tmp_var_5] -> xxtimeab_tmp_var_6_operator/1
  xxtimeab_tmp_var_6_operator/1 -> [timeab_tmp_var_xxtimeab_tmp_var_6]
  [timeab_tmp_var_b] -> xxtimeab_tmp_var_5_operator/2
  [timeab_tmp_var_xxtimeab_tmp_var_4] -> xxtimeab_tmp_var_5_operator/1
  xxtimeab_tmp_var_5_operator/1 -> [timeab_tmp_var_xxtimeab_tmp_var_5]
  [branch_3_xxtimeab_tmp_var_2] -> [branch_3_branch_true_xxtimeab_tmp_var_2]
  [branch_3_branch_true_xxtimeab_tmp_var_2] -> [branch_3_branch_true_xxtimeab_tmp_var_4]
  [branch_3_xxtimeab_tmp_var_3] -> [branch_3_branch_false_xxtimeab_tmp_var_3]
  [branch_3_branch_false_xxtimeab_tmp_var_3] -> [branch_3_branch_false_xxtimeab_tmp_var_4]
  [timeab_tmp_var_xxtimeab_tmp_var_1] -> [branch_3_xxtimeab_tmp_var_1]
  [timeab_tmp_var_xxtimeab_tmp_var_2] -> [branch_3_xxtimeab_tmp_var_2]
  [timeab_tmp_var_xxtimeab_tmp_var_3] -> [branch_3_xxtimeab_tmp_var_3]
  [branch_3_xxtimeab_tmp_var_1] -> branch_3_IF/2
  [branch_3_branch_true_xxtimeab_tmp_var_4] -> branch_3_IF/1
  [branch_3_branch_false_xxtimeab_tmp_var_4] -> branch_3_IF/3
  branch_3_IF/1 -> [branch_3_xxtimeab_tmp_var_4]
  [branch_3_xxtimeab_tmp_var_4] -> [timeab_tmp_var_xxtimeab_tmp_var_4]
  xxtimeab_tmp_var_2_rhs/1 -> [timeab_tmp_var_xxtimeab_tmp_var_2]
  [timeab_tmp_var_a] -> xxtimeab_tmp_var_7_operator/2
  [timeab_tmp_var_internal_clk] -> xxtimeab_tmp_var_7_operator/1
  xxtimeab_tmp_var_7_operator/1 -> [timeab_tmp_var_xxtimeab_tmp_var_7]
  [timeab_tmp_var_b] -> min_call/2(min_b)
  [timeab_tmp_var_xxtimeab_tmp_var_10] -> min_call/1(min_a)
  min_call/1(min_valeur_min) -> [timeab_tmp_var_internal_clk]
  [branch_2_xxtimeab_tmp_var_8] -> [branch_2_branch_true_xxtimeab_tmp_var_8]
  [branch_2_branch_true_xxtimeab_tmp_var_8] -> [branch_2_branch_true_xxtimeab_tmp_var_10]
  [branch_2_xxtimeab_tmp_var_9] -> [branch_2_branch_false_xxtimeab_tmp_var_9]
  [branch_2_branch_false_xxtimeab_tmp_var_9] -> [branch_2_branch_false_xxtimeab_tmp_var_10]
  [timeab_tmp_var_xxtimeab_tmp_var_1] -> [branch_2_xxtimeab_tmp_var_1]
  [timeab_tmp_var_xxtimeab_tmp_var_8] -> [branch_2_xxtimeab_tmp_var_8]
  [timeab_tmp_var_xxtimeab_tmp_var_9] -> [branch_2_xxtimeab_tmp_var_9]
  [branch_2_xxtimeab_tmp_var_1] -> branch_2_IF/2
  [branch_2_branch_true_xxtimeab_tmp_var_10] -> branch_2_IF/1
  [Counter] -> branch_2_IF/3
  branch_2_IF/1 -> [branch_2_xxtimeab_tmp_var_10]
  [branch_2_xxtimeab_tmp_var_10] -> [timeab_tmp_var_xxtimeab_tmp_var_10]
  Arrow_xxtimeab_tmp_var_1_ni_0/1 -> [timeab_tmp_var_xxtimeab_tmp_var_1]
  xxtimeab_tmp_var_1_ni_0_init/1 -> Arrow_xxtimeab_tmp_var_1_ni_0/1
  xxtimeab_tmp_var_8_rhs/1 -> [timeab_tmp_var_xxtimeab_tmp_var_8]
  [timeab_tmp_var_xxtimeab_tmp_var_3] -> xxtimeab_tmp_var_9_operator/2
  xxtimeab_tmp_var_9_rhs_1/1 -> xxtimeab_tmp_var_9_operator/1
  xxtimeab_tmp_var_9_operator/1 -> [timeab_tmp_var_xxtimeab_tmp_var_9]
  [timeab_tmp_var_inside_time_interval] -> timeab_tmp_var_inside_time_interval/1
  [timeab_tmp_var_internal_clk] -> timeab_tmp_var_internal_clk/1
  timeab_tmp_var_b/1 -> [timeab_tmp_var_b]
  timeab_tmp_var_a/1 -> [timeab_tmp_var_a]
  [branch_2_xxtimeab_tmp_var_10] -> counter/1(In1)
  counter/1(Out1) -> [Counter]

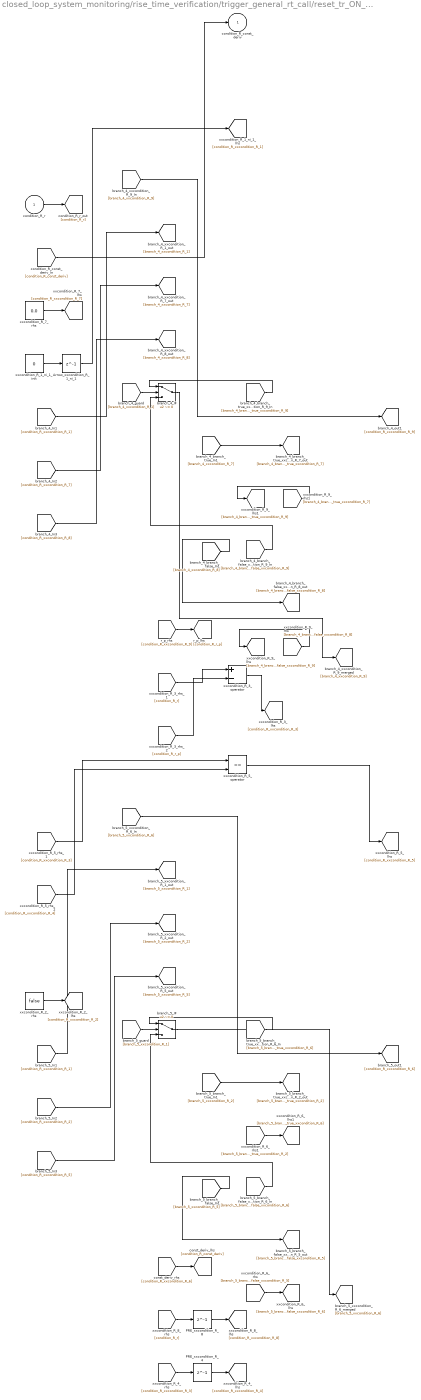
== system closed_loop_system_monitoring/rise_time_verification/trigger_general_rt_call/reset_tr_ON_call/condition_R_call ==
  condition_R_r : Inport  OutDataTypeStr=double
  Arrow_xxcondition_R_1_ni_1 : Delay  DelayLength=1  InitialCondition=1
  PRE_xxcondition_R_4 : Delay  DelayLength=1  InitialCondition=0
  PRE_xxcondition_R_8 : Delay  DelayLength=1  InitialCondition=0
  branch_4_IF : Switch  Criteria=u2 ~= 0  SaturateOnIntegerOverflow=off  InputSameDT=off
  branch_5_IF : Switch  Criteria=u2 ~= 0  SaturateOnIntegerOverflow=off  InputSameDT=off
  xxcondition_R_1_ni_1_init : Constant  Value=0  OutDataTypeStr=boolean
  xxcondition_R_2_rhs : Constant  Value=false  OutDataTypeStr=boolean
  xxcondition_R_3_operator : Sum  Inputs=+-  OutDataTypeStr=double
  xxcondition_R_5_operator : RelationalOperator  Operator===  OutDataTypeStr=boolean  RndMeth=Simplest  InputSameDT=off
  xxcondition_R_7_rhs : Constant  Value=0.0  OutDataTypeStr=double
  condition_R_const_deriv : Outport
  wires:
  PRE_xxcondition_R_4/1 -> [condition_R_xxcondition_R_4]
  [condition_R_xxcondition_R_3] -> PRE_xxcondition_R_4/1
  PRE_xxcondition_R_8/1 -> [condition_R_xxcondition_R_8]
  [condition_R_r] -> PRE_xxcondition_R_8/1
  [condition_R_xxcondition_R_6] -> [condition_R_const_deriv]
  [branch_5_xxcondition_R_2] -> [branch_5_branch_true_xxcondition_R_2]
  [branch_5_branch_true_xxcondition_R_2] -> [branch_5_branch_true_xxcondition_R_6]
  [branch_5_xxcondition_R_5] -> [branch_5_branch_false_xxcondition_R_5]
  [branch_5_branch_false_xxcondition_R_5] -> [branch_5_branch_false_xxcondition_R_6]
  [condition_R_xxcondition_R_1] -> [branch_5_xxcondition_R_1]
  [condition_R_xxcondition_R_2] -> [branch_5_xxcondition_R_2]
  [condition_R_xxcondition_R_5] -> [branch_5_xxcondition_R_5]
  [branch_5_xxcondition_R_1] -> branch_5_IF/2
  [branch_5_branch_true_xxcondition_R_6] -> branch_5_IF/1
  [branch_5_branch_false_xxcondition_R_6] -> branch_5_IF/3
  branch_5_IF/1 -> [branch_5_xxcondition_R_6]
  [branch_5_xxcondition_R_6] -> [condition_R_xxcondition_R_6]
  xxcondition_R_2_rhs/1 -> [condition_R_xxcondition_R_2]
  [condition_R_xxcondition_R_4] -> xxcondition_R_5_operator/2
  [condition_R_xxcondition_R_3] -> xxcondition_R_5_operator/1
  xxcondition_R_5_operator/1 -> [condition_R_xxcondition_R_5]
  [condition_R_r_p] -> xxcondition_R_3_operator/2
  [condition_R_r] -> xxcondition_R_3_operator/1
  xxcondition_R_3_operator/1 -> [condition_R_xxcondition_R_3]
  [condition_R_xxcondition_R_9] -> [condition_R_r_p]
  [branch_4_xxcondition_R_7] -> [branch_4_branch_true_xxcondition_R_7]
  [branch_4_branch_true_xxcondition_R_7] -> [branch_4_branch_true_xxcondition_R_9]
  [branch_4_xxcondition_R_8] -> [branch_4_branch_false_xxcondition_R_8]
  [branch_4_branch_false_xxcondition_R_8] -> [branch_4_branch_false_xxcondition_R_9]
  [condition_R_xxcondition_R_1] -> [branch_4_xxcondition_R_1]
  [condition_R_xxcondition_R_7] -> [branch_4_xxcondition_R_7]
  [condition_R_xxcondition_R_8] -> [branch_4_xxcondition_R_8]
  [branch_4_xxcondition_R_1] -> branch_4_IF/2
  [branch_4_branch_true_xxcondition_R_9] -> branch_4_IF/1
  [branch_4_branch_false_xxcondition_R_9] -> branch_4_IF/3
  branch_4_IF/1 -> [branch_4_xxcondition_R_9]
  [branch_4_xxcondition_R_9] -> [condition_R_xxcondition_R_9]
  Arrow_xxcondition_R_1_ni_1/1 -> [condition_R_xxcondition_R_1]
  xxcondition_R_1_ni_1_init/1 -> Arrow_xxcondition_R_1_ni_1/1
  xxcondition_R_7_rhs/1 -> [condition_R_xxcondition_R_7]
  [condition_R_const_deriv] -> condition_R_const_deriv/1
  condition_R_r/1 -> [condition_R_r]

== system closed_loop_system_monitoring/rise_time_verification/eventually_false_var_call/timeab_var_call/timeab_tmp_var_call/counter ==
  In1 : Inport
  Add : Sum
  Constant : Constant
  Unit Delay : UnitDelay  SampleTime=-1  HasFrameUpgradeWarning=on
  Out1 : Outport
  wires:
  In1/1 -> Unit Delay/1
  Add/1 -> Out1/1
  Constant/1 -> Add/1
  Unit Delay/1 -> Add/2

== system closed_loop_system_monitoring/rise_time_verification/eventually_false_var_call/timeab_var_call/timeab_tmp_var_call/min_call ==
  min_a : Inport
  min_b : Inport  Port=2
  branch_1_IF : Switch  Criteria=u2 ~= 0  SaturateOnIntegerOverflow=off  InputSameDT=off
  xxmin_1_operator : RelationalOperator  Operator=<=  OutDataTypeStr=boolean  RndMeth=Simplest  InputSameDT=off
  min_valeur_min : Outport
  wires:
  min_a/1 -> [min_a]
  min_b/1 -> [min_b]
  [min_valeur_min] -> min_valeur_min/1
  xxmin_1_operator/1 -> [min_xxmin_1]
  [min_a] -> xxmin_1_operator/1
  [min_b] -> xxmin_1_operator/2
  [branch_1_valeur_min] -> [min_valeur_min]
  branch_1_IF/1 -> [branch_1_valeur_min]
  [branch_1_branch_false_valeur_min] -> branch_1_IF/3
  [branch_1_branch_true_valeur_min] -> branch_1_IF/1
  [branch_1_xxmin_1] -> branch_1_IF/2
  [min_b] -> [branch_1_b]
  [min_a] -> [branch_1_a]
  [min_xxmin_1] -> [branch_1_xxmin_1]
  [branch_1_branch_false_b] -> [branch_1_branch_false_valeur_min]
  [branch_1_b] -> [branch_1_branch_false_b]
  [branch_1_branch_true_a] -> [branch_1_branch_true_valeur_min]
  [branch_1_a] -> [branch_1_branch_true_a]

== system closed_loop_system_monitoring/rise_time_verification/eventually_true_var_call/timeab_var_call/timeab_tmp_var_call/counter ==
  In1 : Inport
  Add : Sum
  Constant : Constant
  Unit Delay : UnitDelay  SampleTime=-1  HasFrameUpgradeWarning=on
  Out1 : Outport
  wires:
  In1/1 -> Unit Delay/1
  Add/1 -> Out1/1
  Constant/1 -> Add/1
  Unit Delay/1 -> Add/2

== system closed_loop_system_monitoring/rise_time_verification/eventually_true_var_call/timeab_var_call/timeab_tmp_var_call/min_call ==
  min_a : Inport
  min_b : Inport  Port=2
  branch_1_IF : Switch  Criteria=u2 ~= 0  SaturateOnIntegerOverflow=off  InputSameDT=off
  xxmin_1_operator : RelationalOperator  Operator=<=  OutDataTypeStr=boolean  RndMeth=Simplest  InputSameDT=off
  min_valeur_min : Outport
  wires:
  min_a/1 -> [min_a]
  min_b/1 -> [min_b]
  [min_valeur_min] -> min_valeur_min/1
  xxmin_1_operator/1 -> [min_xxmin_1]
  [min_a] -> xxmin_1_operator/1
  [min_b] -> xxmin_1_operator/2
  [branch_1_valeur_min] -> [min_valeur_min]
  branch_1_IF/1 -> [branch_1_valeur_min]
  [branch_1_branch_false_valeur_min] -> branch_1_IF/3
  [branch_1_branch_true_valeur_min] -> branch_1_IF/1
  [branch_1_xxmin_1] -> branch_1_IF/2
  [min_b] -> [branch_1_b]
  [min_a] -> [branch_1_a]
  [min_xxmin_1] -> [branch_1_xxmin_1]
  [branch_1_branch_false_b] -> [branch_1_branch_false_valeur_min]
  [branch_1_b] -> [branch_1_branch_false_b]
  [branch_1_branch_true_a] -> [branch_1_branch_true_valeur_min]
  [branch_1_a] -> [branch_1_branch_true_a]
